simulink model "test_180429_20K"  (R2018b)
settings: Solver=VariableStepAuto  StartTime=0.0  StopTime=10.0  RelTol=1e-3
values from neighbouring files (symbols this model uses):
  sys1 = sys1_exp    [check_exportvsmake.m]    (also in sumcon2mdlconst_typeA.m = sus.ss)
settings Model: Creator=miyo  LastModifiedBy=miyo

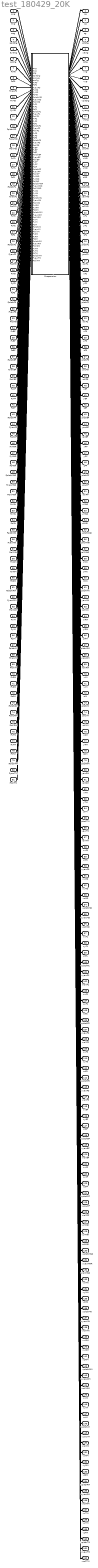
== system test_180429_20K ==
  axg : Inport
  ayg : Inport  Port=2
  azg : Inport  Port=3
  apitchg : Inport  Port=4
  ayawg : Inport  Port=5
  arollg : Inport  Port=6
  FxF0 : Inport  Port=7
  FzF0 : Inport  Port=8
  FyawF0 : Inport  Port=9
  FxMD : Inport  Port=10
  FyMD : Inport  Port=11
  FzMD : Inport  Port=12
  FpitchMD : Inport  Port=13
  FyawMD : Inport  Port=14
  FrollMD : Inport  Port=15
  FxF1 : Inport  Port=16
  FyF1 : Inport  Port=17
  FzF1 : Inport  Port=18
  FpitchF1 : Inport  Port=19
  FyawF1 : Inport  Port=20
  FrollF1 : Inport  Port=21
  FxF2 : Inport  Port=22
  FyF2 : Inport  Port=23
  FzF2 : Inport  Port=24
  FpitchF2 : Inport  Port=25
  FyawF2 : Inport  Port=26
  FrollF2 : Inport  Port=27
  FxF3 : Inport  Port=28
  FyF3 : Inport  Port=29
  FzF3 : Inport  Port=30
  FpitchF3 : Inport  Port=31
  FyawF3 : Inport  Port=32
  FrollF3 : Inport  Port=33
  FxBF : Inport  Port=34
  FyBF : Inport  Port=35
  FzBF : Inport  Port=36
  FpitchBF : Inport  Port=37
  FyawBF : Inport  Port=38
  FrollBF : Inport  Port=39
  FxPF : Inport  Port=40
  FyPF : Inport  Port=41
  FzPF : Inport  Port=42
  FpitchPF : Inport  Port=43
  FyawPF : Inport  Port=44
  FrollPF : Inport  Port=45
  FxMNR : Inport  Port=46
  FyMNR : Inport  Port=47
  FzMNR : Inport  Port=48
  FpitchMNR : Inport  Port=49
  FyawMNR : Inport  Port=50
  FrollMNR : Inport  Port=51
  FxMN : Inport  Port=52
  FyMN : Inport  Port=53
  FzMN : Inport  Port=54
  FpitchMN : Inport  Port=55
  FyawMN : Inport  Port=56
  FrollMN : Inport  Port=57
  FxIRM : Inport  Port=58
  FyIRM : Inport  Port=59
  FzIRM : Inport  Port=60
  FpitchIRM : Inport  Port=61
  FyawIRM : Inport  Port=62
  FrollIRM : Inport  Port=63
  FxIM : Inport  Port=64
  FyIM : Inport  Port=65
  FzIM : Inport  Port=66
  FpitchIM : Inport  Port=67
  FyawIM : Inport  Port=68
  FrollIM : Inport  Port=69
  FxRM : Inport  Port=70
  FyRM : Inport  Port=71
  FzRM : Inport  Port=72
  FpitchRM : Inport  Port=73
  FyawRM : Inport  Port=74
  FrollRM : Inport  Port=75
  FxTM : Inport  Port=76
  FyTM : Inport  Port=77
  FzTM : Inport  Port=78
  FpitchTM : Inport  Port=79
  FyawTM : Inport  Port=80
  FrollTM : Inport  Port=81
  Suspension : Subsystem
  xg : Outport
  yg : Outport  Port=2
  zg : Outport  Port=3
  pitchg : Outport  Port=4
  yawg : Outport  Port=5
  rollg : Outport  Port=6
  vxg : Outport  Port=7
  vyg : Outport  Port=8
  vzg : Outport  Port=9
  vpitchg : Outport  Port=10
  vyawg : Outport  Port=11
  vrollg : Outport  Port=12
  xF0 : Outport  Port=13
  zF0 : Outport  Port=14
  yawF0 : Outport  Port=15
  xMD : Outport  Port=16
  yMD : Outport  Port=17
  zMD : Outport  Port=18
  pitchMD : Outport  Port=19
  yawMD : Outport  Port=20
  rollMD : Outport  Port=21
  xF1 : Outport  Port=22
  yF1 : Outport  Port=23
  zF1 : Outport  Port=24
  pitchF1 : Outport  Port=25
  yawF1 : Outport  Port=26
  rollF1 : Outport  Port=27
  xF2 : Outport  Port=28
  yF2 : Outport  Port=29
  zF2 : Outport  Port=30
  pitchF2 : Outport  Port=31
  yawF2 : Outport  Port=32
  rollF2 : Outport  Port=33
  xF3 : Outport  Port=34
  yF3 : Outport  Port=35
  zF3 : Outport  Port=36
  pitchF3 : Outport  Port=37
  yawF3 : Outport  Port=38
  rollF3 : Outport  Port=39
  xBF : Outport  Port=40
  yBF : Outport  Port=41
  zBF : Outport  Port=42
  pitchBF : Outport  Port=43
  yawBF : Outport  Port=44
  rollBF : Outport  Port=45
  xPF : Outport  Port=46
  yPF : Outport  Port=47
  zPF : Outport  Port=48
  pitchPF : Outport  Port=49
  yawPF : Outport  Port=50
  rollPF : Outport  Port=51
  xMNR : Outport  Port=52
  yMNR : Outport  Port=53
  zMNR : Outport  Port=54
  pitchMNR : Outport  Port=55
  yawMNR : Outport  Port=56
  rollMNR : Outport  Port=57
  xMN : Outport  Port=58
  yMN : Outport  Port=59
  zMN : Outport  Port=60
  pitchMN : Outport  Port=61
  yawMN : Outport  Port=62
  rollMN : Outport  Port=63
  xIRM : Outport  Port=64
  yIRM : Outport  Port=65
  zIRM : Outport  Port=66
  pitchIRM : Outport  Port=67
  yawIRM : Outport  Port=68
  rollIRM : Outport  Port=69
  xIM : Outport  Port=70
  yIM : Outport  Port=71
  zIM : Outport  Port=72
  pitchIM : Outport  Port=73
  yawIM : Outport  Port=74
  rollIM : Outport  Port=75
  xRM : Outport  Port=76
  yRM : Outport  Port=77
  zRM : Outport  Port=78
  pitchRM : Outport  Port=79
  yawRM : Outport  Port=80
  rollRM : Outport  Port=81
  xTM : Outport  Port=82
  yTM : Outport  Port=83
  zTM : Outport  Port=84
  pitchTM : Outport  Port=85
  yawTM : Outport  Port=86
  rollTM : Outport  Port=87
  vxF0 : Outport  Port=88
  vzF0 : Outport  Port=89
  vyawF0 : Outport  Port=90
  vxMD : Outport  Port=91
  vyMD : Outport  Port=92
  vzMD : Outport  Port=93
  vpitchMD : Outport  Port=94
  vyawMD : Outport  Port=95
  vrollMD : Outport  Port=96
  vxF1 : Outport  Port=97
  vyF1 : Outport  Port=98
  vzF1 : Outport  Port=99
  vpitchF1 : Outport  Port=100
  vyawF1 : Outport  Port=101
  vrollF1 : Outport  Port=102
  vxF2 : Outport  Port=103
  vyF2 : Outport  Port=104
  vzF2 : Outport  Port=105
  vpitchF2 : Outport  Port=106
  vyawF2 : Outport  Port=107
  vrollF2 : Outport  Port=108
  vxF3 : Outport  Port=109
  vyF3 : Outport  Port=110
  vzF3 : Outport  Port=111
  vpitchF3 : Outport  Port=112
  vyawF3 : Outport  Port=113
  vrollF3 : Outport  Port=114
  vxBF : Outport  Port=115
  vyBF : Outport  Port=116
  vzBF : Outport  Port=117
  vpitchBF : Outport  Port=118
  vyawBF : Outport  Port=119
  vrollBF : Outport  Port=120
  vxPF : Outport  Port=121
  vyPF : Outport  Port=122
  vzPF : Outport  Port=123
  vpitchPF : Outport  Port=124
  vyawPF : Outport  Port=125
  vrollPF : Outport  Port=126
  vxMNR : Outport  Port=127
  vyMNR : Outport  Port=128
  vzMNR : Outport  Port=129
  vpitchMNR : Outport  Port=130
  vyawMNR : Outport  Port=131
  vrollMNR : Outport  Port=132
  vxMN : Outport  Port=133
  vyMN : Outport  Port=134
  vzMN : Outport  Port=135
  vpitchMN : Outport  Port=136
  vyawMN : Outport  Port=137
  vrollMN : Outport  Port=138
  vxIRM : Outport  Port=139
  vyIRM : Outport  Port=140
  vzIRM : Outport  Port=141
  vpitchIRM : Outport  Port=142
  vyawIRM : Outport  Port=143
  vrollIRM : Outport  Port=144
  vxIM : Outport  Port=145
  vyIM : Outport  Port=146
  vzIM : Outport  Port=147
  vpitchIM : Outport  Port=148
  vyawIM : Outport  Port=149
  vrollIM : Outport  Port=150
  vxRM : Outport  Port=151
  vyRM : Outport  Port=152
  vzRM : Outport  Port=153
  vpitchRM : Outport  Port=154
  vyawRM : Outport  Port=155
  vrollRM : Outport  Port=156
  vxTM : Outport  Port=157
  vyTM : Outport  Port=158
  vzTM : Outport  Port=159
  vpitchTM : Outport  Port=160
  vyawTM : Outport  Port=161
  vrollTM : Outport  Port=162
  wires:
  axg/1 -> Suspension/1(axg)
  ayg/1 -> Suspension/2(ayg)
  azg/1 -> Suspension/3(azg)
  apitchg/1 -> Suspension/4(apitchg)
  ayawg/1 -> Suspension/5(ayawg)
  arollg/1 -> Suspension/6(arollg)
  FxF0/1 -> Suspension/7(FxF0)
  FzF0/1 -> Suspension/8(FzF0)
  FyawF0/1 -> Suspension/9(FyawF0)
  FxMD/1 -> Suspension/10(FxMD)
  FyMD/1 -> Suspension/11(FyMD)
  FzMD/1 -> Suspension/12(FzMD)
  FpitchMD/1 -> Suspension/13(FpitchMD)
  FyawMD/1 -> Suspension/14(FyawMD)
  FrollMD/1 -> Suspension/15(FrollMD)
  FxF1/1 -> Suspension/16(FxF1)
  FyF1/1 -> Suspension/17(FyF1)
  FzF1/1 -> Suspension/18(FzF1)
  FpitchF1/1 -> Suspension/19(FpitchF1)
  FyawF1/1 -> Suspension/20(FyawF1)
  FrollF1/1 -> Suspension/21(FrollF1)
  FxF2/1 -> Suspension/22(FxF2)
  FyF2/1 -> Suspension/23(FyF2)
  FzF2/1 -> Suspension/24(FzF2)
  FpitchF2/1 -> Suspension/25(FpitchF2)
  FyawF2/1 -> Suspension/26(FyawF2)
  FrollF2/1 -> Suspension/27(FrollF2)
  FxF3/1 -> Suspension/28(FxF3)
  FyF3/1 -> Suspension/29(FyF3)
  FzF3/1 -> Suspension/30(FzF3)
  FpitchF3/1 -> Suspension/31(FpitchF3)
  FyawF3/1 -> Suspension/32(FyawF3)
  FrollF3/1 -> Suspension/33(FrollF3)
  FxBF/1 -> Suspension/34(FxBF)
  FyBF/1 -> Suspension/35(FyBF)
  FzBF/1 -> Suspension/36(FzBF)
  FpitchBF/1 -> Suspension/37(FpitchBF)
  FyawBF/1 -> Suspension/38(FyawBF)
  FrollBF/1 -> Suspension/39(FrollBF)
  FxPF/1 -> Suspension/40(FxPF)
  FyPF/1 -> Suspension/41(FyPF)
  FzPF/1 -> Suspension/42(FzPF)
  FpitchPF/1 -> Suspension/43(FpitchPF)
  FyawPF/1 -> Suspension/44(FyawPF)
  FrollPF/1 -> Suspension/45(FrollPF)
  FxMNR/1 -> Suspension/46(FxMNR)
  FyMNR/1 -> Suspension/47(FyMNR)
  FzMNR/1 -> Suspension/48(FzMNR)
  FpitchMNR/1 -> Suspension/49(FpitchMNR)
  FyawMNR/1 -> Suspension/50(FyawMNR)
  FrollMNR/1 -> Suspension/51(FrollMNR)
  FxMN/1 -> Suspension/52(FxMN)
  FyMN/1 -> Suspension/53(FyMN)
  FzMN/1 -> Suspension/54(FzMN)
  FpitchMN/1 -> Suspension/55(FpitchMN)
  FyawMN/1 -> Suspension/56(FyawMN)
  FrollMN/1 -> Suspension/57(FrollMN)
  FxIRM/1 -> Suspension/58(FxIRM)
  FyIRM/1 -> Suspension/59(FyIRM)
  FzIRM/1 -> Suspension/60(FzIRM)
  FpitchIRM/1 -> Suspension/61(FpitchIRM)
  FyawIRM/1 -> Suspension/62(FyawIRM)
  FrollIRM/1 -> Suspension/63(FrollIRM)
  FxIM/1 -> Suspension/64(FxIM)
  FyIM/1 -> Suspension/65(FyIM)
  FzIM/1 -> Suspension/66(FzIM)
  FpitchIM/1 -> Suspension/67(FpitchIM)
  FyawIM/1 -> Suspension/68(FyawIM)
  FrollIM/1 -> Suspension/69(FrollIM)
  FxRM/1 -> Suspension/70(FxRM)
  FyRM/1 -> Suspension/71(FyRM)
  FzRM/1 -> Suspension/72(FzRM)
  FpitchRM/1 -> Suspension/73(FpitchRM)
  FyawRM/1 -> Suspension/74(FyawRM)
  FrollRM/1 -> Suspension/75(FrollRM)
  FxTM/1 -> Suspension/76(FxTM)
  FyTM/1 -> Suspension/77(FyTM)
  FzTM/1 -> Suspension/78(FzTM)
  FpitchTM/1 -> Suspension/79(FpitchTM)
  FyawTM/1 -> Suspension/80(FyawTM)
  FrollTM/1 -> Suspension/81(FrollTM)
  Suspension/1(xg) -> xg/1
  Suspension/2(yg) -> yg/1
  Suspension/3(zg) -> zg/1
  Suspension/4(pitchg) -> pitchg/1
  Suspension/5(yawg) -> yawg/1
  Suspension/6(rollg) -> rollg/1
  Suspension/7(vxg) -> vxg/1
  Suspension/8(vyg) -> vyg/1
  Suspension/9(vzg) -> vzg/1
  Suspension/10(vpitchg) -> vpitchg/1
  Suspension/11(vyawg) -> vyawg/1
  Suspension/12(vrollg) -> vrollg/1
  Suspension/13(xF0) -> xF0/1
  Suspension/14(zF0) -> zF0/1
  Suspension/15(yawF0) -> yawF0/1
  Suspension/16(xMD) -> xMD/1
  Suspension/17(yMD) -> yMD/1
  Suspension/18(zMD) -> zMD/1
  Suspension/19(pitchMD) -> pitchMD/1
  Suspension/20(yawMD) -> yawMD/1
  Suspension/21(rollMD) -> rollMD/1
  Suspension/22(xF1) -> xF1/1
  Suspension/23(yF1) -> yF1/1
  Suspension/24(zF1) -> zF1/1
  Suspension/25(pitchF1) -> pitchF1/1
  Suspension/26(yawF1) -> yawF1/1
  Suspension/27(rollF1) -> rollF1/1
  Suspension/28(xF2) -> xF2/1
  Suspension/29(yF2) -> yF2/1
  Suspension/30(zF2) -> zF2/1
  Suspension/31(pitchF2) -> pitchF2/1
  Suspension/32(yawF2) -> yawF2/1
  Suspension/33(rollF2) -> rollF2/1
  Suspension/34(xF3) -> xF3/1
  Suspension/35(yF3) -> yF3/1
  Suspension/36(zF3) -> zF3/1
  Suspension/37(pitchF3) -> pitchF3/1
  Suspension/38(yawF3) -> yawF3/1
  Suspension/39(rollF3) -> rollF3/1
  Suspension/40(xBF) -> xBF/1
  Suspension/41(yBF) -> yBF/1
  Suspension/42(zBF) -> zBF/1
  Suspension/43(pitchBF) -> pitchBF/1
  Suspension/44(yawBF) -> yawBF/1
  Suspension/45(rollBF) -> rollBF/1
  Suspension/46(xPF) -> xPF/1
  Suspension/47(yPF) -> yPF/1
  Suspension/48(zPF) -> zPF/1
  Suspension/49(pitchPF) -> pitchPF/1
  Suspension/50(yawPF) -> yawPF/1
  Suspension/51(rollPF) -> rollPF/1
  Suspension/52(xMNR) -> xMNR/1
  Suspension/53(yMNR) -> yMNR/1
  Suspension/54(zMNR) -> zMNR/1
  Suspension/55(pitchMNR) -> pitchMNR/1
  Suspension/56(yawMNR) -> yawMNR/1
  Suspension/57(rollMNR) -> rollMNR/1
  Suspension/58(xMN) -> xMN/1
  Suspension/59(yMN) -> yMN/1
  Suspension/60(zMN) -> zMN/1
  Suspension/61(pitchMN) -> pitchMN/1
  Suspension/62(yawMN) -> yawMN/1
  Suspension/63(rollMN) -> rollMN/1
  Suspension/64(xIRM) -> xIRM/1
  Suspension/65(yIRM) -> yIRM/1
  Suspension/66(zIRM) -> zIRM/1
  Suspension/67(pitchIRM) -> pitchIRM/1
  Suspension/68(yawIRM) -> yawIRM/1
  Suspension/69(rollIRM) -> rollIRM/1
  Suspension/70(xIM) -> xIM/1
  Suspension/71(yIM) -> yIM/1
  Suspension/72(zIM) -> zIM/1
  Suspension/73(pitchIM) -> pitchIM/1
  Suspension/74(yawIM) -> yawIM/1
  Suspension/75(rollIM) -> rollIM/1
  Suspension/76(xRM) -> xRM/1
  Suspension/77(yRM) -> yRM/1
  Suspension/78(zRM) -> zRM/1
  Suspension/79(pitchRM) -> pitchRM/1
  Suspension/80(yawRM) -> yawRM/1
  Suspension/81(rollRM) -> rollRM/1
  Suspension/82(xTM) -> xTM/1
  Suspension/83(yTM) -> yTM/1
  Suspension/84(zTM) -> zTM/1
  Suspension/85(pitchTM) -> pitchTM/1
  Suspension/86(yawTM) -> yawTM/1
  Suspension/87(rollTM) -> rollTM/1
  Suspension/88(vxF0) -> vxF0/1
  Suspension/89(vzF0) -> vzF0/1
  Suspension/90(vyawF0) -> vyawF0/1
  Suspension/91(vxMD) -> vxMD/1
  Suspension/92(vyMD) -> vyMD/1
  Suspension/93(vzMD) -> vzMD/1
  Suspension/94(vpitchMD) -> vpitchMD/1
  Suspension/95(vyawMD) -> vyawMD/1
  Suspension/96(vrollMD) -> vrollMD/1
  Suspension/97(vxF1) -> vxF1/1
  Suspension/98(vyF1) -> vyF1/1
  Suspension/99(vzF1) -> vzF1/1
  Suspension/100(vpitchF1) -> vpitchF1/1
  Suspension/101(vyawF1) -> vyawF1/1
  Suspension/102(vrollF1) -> vrollF1/1
  Suspension/103(vxF2) -> vxF2/1
  Suspension/104(vyF2) -> vyF2/1
  Suspension/105(vzF2) -> vzF2/1
  Suspension/106(vpitchF2) -> vpitchF2/1
  Suspension/107(vyawF2) -> vyawF2/1
  Suspension/108(vrollF2) -> vrollF2/1
  Suspension/109(vxF3) -> vxF3/1
  Suspension/110(vyF3) -> vyF3/1
  Suspension/111(vzF3) -> vzF3/1
  Suspension/112(vpitchF3) -> vpitchF3/1
  Suspension/113(vyawF3) -> vyawF3/1
  Suspension/114(vrollF3) -> vrollF3/1
  Suspension/115(vxBF) -> vxBF/1
  Suspension/116(vyBF) -> vyBF/1
  Suspension/117(vzBF) -> vzBF/1
  Suspension/118(vpitchBF) -> vpitchBF/1
  Suspension/119(vyawBF) -> vyawBF/1
  Suspension/120(vrollBF) -> vrollBF/1
  Suspension/121(vxPF) -> vxPF/1
  Suspension/122(vyPF) -> vyPF/1
  Suspension/123(vzPF) -> vzPF/1
  Suspension/124(vpitchPF) -> vpitchPF/1
  Suspension/125(vyawPF) -> vyawPF/1
  Suspension/126(vrollPF) -> vrollPF/1
  Suspension/127(vxMNR) -> vxMNR/1
  Suspension/128(vyMNR) -> vyMNR/1
  Suspension/129(vzMNR) -> vzMNR/1
  Suspension/130(vpitchMNR) -> vpitchMNR/1
  Suspension/131(vyawMNR) -> vyawMNR/1
  Suspension/132(vrollMNR) -> vrollMNR/1
  Suspension/133(vxMN) -> vxMN/1
  Suspension/134(vyMN) -> vyMN/1
  Suspension/135(vzMN) -> vzMN/1
  Suspension/136(vpitchMN) -> vpitchMN/1
  Suspension/137(vyawMN) -> vyawMN/1
  Suspension/138(vrollMN) -> vrollMN/1
  Suspension/139(vxIRM) -> vxIRM/1
  Suspension/140(vyIRM) -> vyIRM/1
  Suspension/141(vzIRM) -> vzIRM/1
  Suspension/142(vpitchIRM) -> vpitchIRM/1
  Suspension/143(vyawIRM) -> vyawIRM/1
  Suspension/144(vrollIRM) -> vrollIRM/1
  Suspension/145(vxIM) -> vxIM/1
  Suspension/146(vyIM) -> vyIM/1
  Suspension/147(vzIM) -> vzIM/1
  Suspension/148(vpitchIM) -> vpitchIM/1
  Suspension/149(vyawIM) -> vyawIM/1
  Suspension/150(vrollIM) -> vrollIM/1
  Suspension/151(vxRM) -> vxRM/1
  Suspension/152(vyRM) -> vyRM/1
  Suspension/153(vzRM) -> vzRM/1
  Suspension/154(vpitchRM) -> vpitchRM/1
  Suspension/155(vyawRM) -> vyawRM/1
  Suspension/156(vrollRM) -> vrollRM/1
  Suspension/157(vxTM) -> vxTM/1
  Suspension/158(vyTM) -> vyTM/1
  Suspension/159(vzTM) -> vzTM/1
  Suspension/160(vpitchTM) -> vpitchTM/1
  Suspension/161(vyawTM) -> vyawTM/1
  Suspension/162(vrollTM) -> vrollTM/1

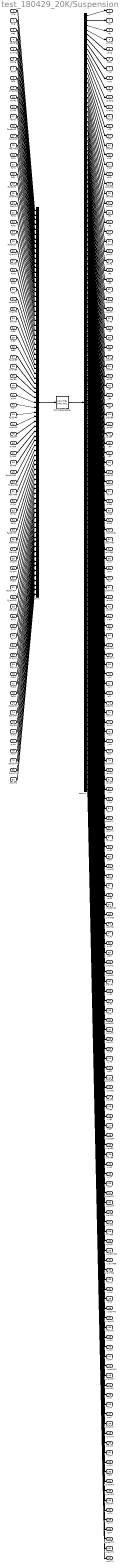
== system test_180429_20K/Suspension ==
  axg : Inport
  ayg : Inport  Port=2
  azg : Inport  Port=3
  apitchg : Inport  Port=4
  ayawg : Inport  Port=5
  arollg : Inport  Port=6
  FxF0 : Inport  Port=7
  FzF0 : Inport  Port=8
  FyawF0 : Inport  Port=9
  FxMD : Inport  Port=10
  FyMD : Inport  Port=11
  FzMD : Inport  Port=12
  FpitchMD : Inport  Port=13
  FyawMD : Inport  Port=14
  FrollMD : Inport  Port=15
  FxF1 : Inport  Port=16
  FyF1 : Inport  Port=17
  FzF1 : Inport  Port=18
  FpitchF1 : Inport  Port=19
  FyawF1 : Inport  Port=20
  FrollF1 : Inport  Port=21
  FxF2 : Inport  Port=22
  FyF2 : Inport  Port=23
  FzF2 : Inport  Port=24
  FpitchF2 : Inport  Port=25
  FyawF2 : Inport  Port=26
  FrollF2 : Inport  Port=27
  FxF3 : Inport  Port=28
  FyF3 : Inport  Port=29
  FzF3 : Inport  Port=30
  FpitchF3 : Inport  Port=31
  FyawF3 : Inport  Port=32
  FrollF3 : Inport  Port=33
  FxBF : Inport  Port=34
  FyBF : Inport  Port=35
  FzBF : Inport  Port=36
  FpitchBF : Inport  Port=37
  FyawBF : Inport  Port=38
  FrollBF : Inport  Port=39
  FxPF : Inport  Port=40
  FyPF : Inport  Port=41
  FzPF : Inport  Port=42
  FpitchPF : Inport  Port=43
  FyawPF : Inport  Port=44
  FrollPF : Inport  Port=45
  FxMNR : Inport  Port=46
  FyMNR : Inport  Port=47
  FzMNR : Inport  Port=48
  FpitchMNR : Inport  Port=49
  FyawMNR : Inport  Port=50
  FrollMNR : Inport  Port=51
  FxMN : Inport  Port=52
  FyMN : Inport  Port=53
  FzMN : Inport  Port=54
  FpitchMN : Inport  Port=55
  FyawMN : Inport  Port=56
  FrollMN : Inport  Port=57
  FxIRM : Inport  Port=58
  FyIRM : Inport  Port=59
  FzIRM : Inport  Port=60
  FpitchIRM : Inport  Port=61
  FyawIRM : Inport  Port=62
  FrollIRM : Inport  Port=63
  FxIM : Inport  Port=64
  FyIM : Inport  Port=65
  FzIM : Inport  Port=66
  FpitchIM : Inport  Port=67
  FyawIM : Inport  Port=68
  FrollIM : Inport  Port=69
  FxRM : Inport  Port=70
  FyRM : Inport  Port=71
  FzRM : Inport  Port=72
  FpitchRM : Inport  Port=73
  FyawRM : Inport  Port=74
  FrollRM : Inport  Port=75
  FxTM : Inport  Port=76
  FyTM : Inport  Port=77
  FzTM : Inport  Port=78
  FpitchTM : Inport  Port=79
  FyawTM : Inport  Port=80
  FrollTM : Inport  Port=81
  SAS State-Space : StateSpace  A=sys1.A  B=sys1.B  C=sys1.C  D=sys1.D  InitialCondition=0  ContinuousStateAttributes='SUS_SS_MODEL'
  demux : Demux  Outputs=162
  mux : Mux  Inputs=81
  xg : Outport
  yg : Outport  Port=2
  zg : Outport  Port=3
  pitchg : Outport  Port=4
  yawg : Outport  Port=5
  rollg : Outport  Port=6
  vxg : Outport  Port=7
  vyg : Outport  Port=8
  vzg : Outport  Port=9
  vpitchg : Outport  Port=10
  vyawg : Outport  Port=11
  vrollg : Outport  Port=12
  xF0 : Outport  Port=13
  zF0 : Outport  Port=14
  yawF0 : Outport  Port=15
  xMD : Outport  Port=16
  yMD : Outport  Port=17
  zMD : Outport  Port=18
  pitchMD : Outport  Port=19
  yawMD : Outport  Port=20
  rollMD : Outport  Port=21
  xF1 : Outport  Port=22
  yF1 : Outport  Port=23
  zF1 : Outport  Port=24
  pitchF1 : Outport  Port=25
  yawF1 : Outport  Port=26
  rollF1 : Outport  Port=27
  xF2 : Outport  Port=28
  yF2 : Outport  Port=29
  zF2 : Outport  Port=30
  pitchF2 : Outport  Port=31
  yawF2 : Outport  Port=32
  rollF2 : Outport  Port=33
  xF3 : Outport  Port=34
  yF3 : Outport  Port=35
  zF3 : Outport  Port=36
  pitchF3 : Outport  Port=37
  yawF3 : Outport  Port=38
  rollF3 : Outport  Port=39
  xBF : Outport  Port=40
  yBF : Outport  Port=41
  zBF : Outport  Port=42
  pitchBF : Outport  Port=43
  yawBF : Outport  Port=44
  rollBF : Outport  Port=45
  xPF : Outport  Port=46
  yPF : Outport  Port=47
  zPF : Outport  Port=48
  pitchPF : Outport  Port=49
  yawPF : Outport  Port=50
  rollPF : Outport  Port=51
  xMNR : Outport  Port=52
  yMNR : Outport  Port=53
  zMNR : Outport  Port=54
  pitchMNR : Outport  Port=55
  yawMNR : Outport  Port=56
  rollMNR : Outport  Port=57
  xMN : Outport  Port=58
  yMN : Outport  Port=59
  zMN : Outport  Port=60
  pitchMN : Outport  Port=61
  yawMN : Outport  Port=62
  rollMN : Outport  Port=63
  xIRM : Outport  Port=64
  yIRM : Outport  Port=65
  zIRM : Outport  Port=66
  pitchIRM : Outport  Port=67
  yawIRM : Outport  Port=68
  rollIRM : Outport  Port=69
  xIM : Outport  Port=70
  yIM : Outport  Port=71
  zIM : Outport  Port=72
  pitchIM : Outport  Port=73
  yawIM : Outport  Port=74
  rollIM : Outport  Port=75
  xRM : Outport  Port=76
  yRM : Outport  Port=77
  zRM : Outport  Port=78
  pitchRM : Outport  Port=79
  yawRM : Outport  Port=80
  rollRM : Outport  Port=81
  xTM : Outport  Port=82
  yTM : Outport  Port=83
  zTM : Outport  Port=84
  pitchTM : Outport  Port=85
  yawTM : Outport  Port=86
  rollTM : Outport  Port=87
  vxF0 : Outport  Port=88
  vzF0 : Outport  Port=89
  vyawF0 : Outport  Port=90
  vxMD : Outport  Port=91
  vyMD : Outport  Port=92
  vzMD : Outport  Port=93
  vpitchMD : Outport  Port=94
  vyawMD : Outport  Port=95
  vrollMD : Outport  Port=96
  vxF1 : Outport  Port=97
  vyF1 : Outport  Port=98
  vzF1 : Outport  Port=99
  vpitchF1 : Outport  Port=100
  vyawF1 : Outport  Port=101
  vrollF1 : Outport  Port=102
  vxF2 : Outport  Port=103
  vyF2 : Outport  Port=104
  vzF2 : Outport  Port=105
  vpitchF2 : Outport  Port=106
  vyawF2 : Outport  Port=107
  vrollF2 : Outport  Port=108
  vxF3 : Outport  Port=109
  vyF3 : Outport  Port=110
  vzF3 : Outport  Port=111
  vpitchF3 : Outport  Port=112
  vyawF3 : Outport  Port=113
  vrollF3 : Outport  Port=114
  vxBF : Outport  Port=115
  vyBF : Outport  Port=116
  vzBF : Outport  Port=117
  vpitchBF : Outport  Port=118
  vyawBF : Outport  Port=119
  vrollBF : Outport  Port=120
  vxPF : Outport  Port=121
  vyPF : Outport  Port=122
  vzPF : Outport  Port=123
  vpitchPF : Outport  Port=124
  vyawPF : Outport  Port=125
  vrollPF : Outport  Port=126
  vxMNR : Outport  Port=127
  vyMNR : Outport  Port=128
  vzMNR : Outport  Port=129
  vpitchMNR : Outport  Port=130
  vyawMNR : Outport  Port=131
  vrollMNR : Outport  Port=132
  vxMN : Outport  Port=133
  vyMN : Outport  Port=134
  vzMN : Outport  Port=135
  vpitchMN : Outport  Port=136
  vyawMN : Outport  Port=137
  vrollMN : Outport  Port=138
  vxIRM : Outport  Port=139
  vyIRM : Outport  Port=140
  vzIRM : Outport  Port=141
  vpitchIRM : Outport  Port=142
  vyawIRM : Outport  Port=143
  vrollIRM : Outport  Port=144
  vxIM : Outport  Port=145
  vyIM : Outport  Port=146
  vzIM : Outport  Port=147
  vpitchIM : Outport  Port=148
  vyawIM : Outport  Port=149
  vrollIM : Outport  Port=150
  vxRM : Outport  Port=151
  vyRM : Outport  Port=152
  vzRM : Outport  Port=153
  vpitchRM : Outport  Port=154
  vyawRM : Outport  Port=155
  vrollRM : Outport  Port=156
  vxTM : Outport  Port=157
  vyTM : Outport  Port=158
  vzTM : Outport  Port=159
  vpitchTM : Outport  Port=160
  vyawTM : Outport  Port=161
  vrollTM : Outport  Port=162
  wires:
  mux/1 -> SAS State-Space/1
  SAS State-Space/1 -> demux/1
  axg/1 -> mux/1
  ayg/1 -> mux/2
  azg/1 -> mux/3
  apitchg/1 -> mux/4
  ayawg/1 -> mux/5
  arollg/1 -> mux/6
  FxF0/1 -> mux/7
  FzF0/1 -> mux/8
  FyawF0/1 -> mux/9
  FxMD/1 -> mux/10
  FyMD/1 -> mux/11
  FzMD/1 -> mux/12
  FpitchMD/1 -> mux/13
  FyawMD/1 -> mux/14
  FrollMD/1 -> mux/15
  FxF1/1 -> mux/16
  FyF1/1 -> mux/17
  FzF1/1 -> mux/18
  FpitchF1/1 -> mux/19
  FyawF1/1 -> mux/20
  FrollF1/1 -> mux/21
  FxF2/1 -> mux/22
  FyF2/1 -> mux/23
  FzF2/1 -> mux/24
  FpitchF2/1 -> mux/25
  FyawF2/1 -> mux/26
  FrollF2/1 -> mux/27
  FxF3/1 -> mux/28
  FyF3/1 -> mux/29
  FzF3/1 -> mux/30
  FpitchF3/1 -> mux/31
  FyawF3/1 -> mux/32
  FrollF3/1 -> mux/33
  FxBF/1 -> mux/34
  FyBF/1 -> mux/35
  FzBF/1 -> mux/36
  FpitchBF/1 -> mux/37
  FyawBF/1 -> mux/38
  FrollBF/1 -> mux/39
  FxPF/1 -> mux/40
  FyPF/1 -> mux/41
  FzPF/1 -> mux/42
  FpitchPF/1 -> mux/43
  FyawPF/1 -> mux/44
  FrollPF/1 -> mux/45
  FxMNR/1 -> mux/46
  FyMNR/1 -> mux/47
  FzMNR/1 -> mux/48
  FpitchMNR/1 -> mux/49
  FyawMNR/1 -> mux/50
  FrollMNR/1 -> mux/51
  FxMN/1 -> mux/52
  FyMN/1 -> mux/53
  FzMN/1 -> mux/54
  FpitchMN/1 -> mux/55
  FyawMN/1 -> mux/56
  FrollMN/1 -> mux/57
  FxIRM/1 -> mux/58
  FyIRM/1 -> mux/59
  FzIRM/1 -> mux/60
  FpitchIRM/1 -> mux/61
  FyawIRM/1 -> mux/62
  FrollIRM/1 -> mux/63
  FxIM/1 -> mux/64
  FyIM/1 -> mux/65
  FzIM/1 -> mux/66
  FpitchIM/1 -> mux/67
  FyawIM/1 -> mux/68
  FrollIM/1 -> mux/69
  FxRM/1 -> mux/70
  FyRM/1 -> mux/71
  FzRM/1 -> mux/72
  FpitchRM/1 -> mux/73
  FyawRM/1 -> mux/74
  FrollRM/1 -> mux/75
  FxTM/1 -> mux/76
  FyTM/1 -> mux/77
  FzTM/1 -> mux/78
  FpitchTM/1 -> mux/79
  FyawTM/1 -> mux/80
  FrollTM/1 -> mux/81
  demux/1 -> xg/1
  demux/2 -> yg/1
  demux/3 -> zg/1
  demux/4 -> pitchg/1
  demux/5 -> yawg/1
  demux/6 -> rollg/1
  demux/7 -> vxg/1
  demux/8 -> vyg/1
  demux/9 -> vzg/1
  demux/10 -> vpitchg/1
  demux/11 -> vyawg/1
  demux/12 -> vrollg/1
  demux/13 -> xF0/1
  demux/14 -> zF0/1
  demux/15 -> yawF0/1
  demux/16 -> xMD/1
  demux/17 -> yMD/1
  demux/18 -> zMD/1
  demux/19 -> pitchMD/1
  demux/20 -> yawMD/1
  demux/21 -> rollMD/1
  demux/22 -> xF1/1
  demux/23 -> yF1/1
  demux/24 -> zF1/1
  demux/25 -> pitchF1/1
  demux/26 -> yawF1/1
  demux/27 -> rollF1/1
  demux/28 -> xF2/1
  demux/29 -> yF2/1
  demux/30 -> zF2/1
  demux/31 -> pitchF2/1
  demux/32 -> yawF2/1
  demux/33 -> rollF2/1
  demux/34 -> xF3/1
  demux/35 -> yF3/1
  demux/36 -> zF3/1
  demux/37 -> pitchF3/1
  demux/38 -> yawF3/1
  demux/39 -> rollF3/1
  demux/40 -> xBF/1
  demux/41 -> yBF/1
  demux/42 -> zBF/1
  demux/43 -> pitchBF/1
  demux/44 -> yawBF/1
  demux/45 -> rollBF/1
  demux/46 -> xPF/1
  demux/47 -> yPF/1
  demux/48 -> zPF/1
  demux/49 -> pitchPF/1
  demux/50 -> yawPF/1
  demux/51 -> rollPF/1
  demux/52 -> xMNR/1
  demux/53 -> yMNR/1
  demux/54 -> zMNR/1
  demux/55 -> pitchMNR/1
  demux/56 -> yawMNR/1
  demux/57 -> rollMNR/1
  demux/58 -> xMN/1
  demux/59 -> yMN/1
  demux/60 -> zMN/1
  demux/61 -> pitchMN/1
  demux/62 -> yawMN/1
  demux/63 -> rollMN/1
  demux/64 -> xIRM/1
  demux/65 -> yIRM/1
  demux/66 -> zIRM/1
  demux/67 -> pitchIRM/1
  demux/68 -> yawIRM/1
  demux/69 -> rollIRM/1
  demux/70 -> xIM/1
  demux/71 -> yIM/1
  demux/72 -> zIM/1
  demux/73 -> pitchIM/1
  demux/74 -> yawIM/1
  demux/75 -> rollIM/1
  demux/76 -> xRM/1
  demux/77 -> yRM/1
  demux/78 -> zRM/1
  demux/79 -> pitchRM/1
  demux/80 -> yawRM/1
  demux/81 -> rollRM/1
  demux/82 -> xTM/1
  demux/83 -> yTM/1
  demux/84 -> zTM/1
  demux/85 -> pitchTM/1
  demux/86 -> yawTM/1
  demux/87 -> rollTM/1
  demux/88 -> vxF0/1
  demux/89 -> vzF0/1
  demux/90 -> vyawF0/1
  demux/91 -> vxMD/1
  demux/92 -> vyMD/1
  demux/93 -> vzMD/1
  demux/94 -> vpitchMD/1
  demux/95 -> vyawMD/1
  demux/96 -> vrollMD/1
  demux/97 -> vxF1/1
  demux/98 -> vyF1/1
  demux/99 -> vzF1/1
  demux/100 -> vpitchF1/1
  demux/101 -> vyawF1/1
  demux/102 -> vrollF1/1
  demux/103 -> vxF2/1
  demux/104 -> vyF2/1
  demux/105 -> vzF2/1
  demux/106 -> vpitchF2/1
  demux/107 -> vyawF2/1
  demux/108 -> vrollF2/1
  demux/109 -> vxF3/1
  demux/110 -> vyF3/1
  demux/111 -> vzF3/1
  demux/112 -> vpitchF3/1
  demux/113 -> vyawF3/1
  demux/114 -> vrollF3/1
  demux/115 -> vxBF/1
  demux/116 -> vyBF/1
  demux/117 -> vzBF/1
  demux/118 -> vpitchBF/1
  demux/119 -> vyawBF/1
  demux/120 -> vrollBF/1
  demux/121 -> vxPF/1
  demux/122 -> vyPF/1
  demux/123 -> vzPF/1
  demux/124 -> vpitchPF/1
  demux/125 -> vyawPF/1
  demux/126 -> vrollPF/1
  demux/127 -> vxMNR/1
  demux/128 -> vyMNR/1
  demux/129 -> vzMNR/1
  demux/130 -> vpitchMNR/1
  demux/131 -> vyawMNR/1
  demux/132 -> vrollMNR/1
  demux/133 -> vxMN/1
  demux/134 -> vyMN/1
  demux/135 -> vzMN/1
  demux/136 -> vpitchMN/1
  demux/137 -> vyawMN/1
  demux/138 -> vrollMN/1
  demux/139 -> vxIRM/1
  demux/140 -> vyIRM/1
  demux/141 -> vzIRM/1
  demux/142 -> vpitchIRM/1
  demux/143 -> vyawIRM/1
  demux/144 -> vrollIRM/1
  demux/145 -> vxIM/1
  demux/146 -> vyIM/1
  demux/147 -> vzIM/1
  demux/148 -> vpitchIM/1
  demux/149 -> vyawIM/1
  demux/150 -> vrollIM/1
  demux/151 -> vxRM/1
  demux/152 -> vyRM/1
  demux/153 -> vzRM/1
  demux/154 -> vpitchRM/1
  demux/155 -> vyawRM/1
  demux/156 -> vrollRM/1
  demux/157 -> vxTM/1
  demux/158 -> vyTM/1
  demux/159 -> vzTM/1
  demux/160 -> vpitchTM/1
  demux/161 -> vyawTM/1
  demux/162 -> vrollTM/1
